simulink subsystem "Encoder_balrob"  (R2024b)
settings: Solver=VariableStepAuto  StartTime=0.0  StopTime=10.0  RelTol=1e-3
values from neighbouring files (symbols this model uses):
  Ts = 1e-2    (= 0.01)    [Plant_balrob_params.m]
undefined symbols (not defined in the file or in its folder): gbox, sens
settings Model: Creator=federico  LastModifiedBy=Riccardo Grosso

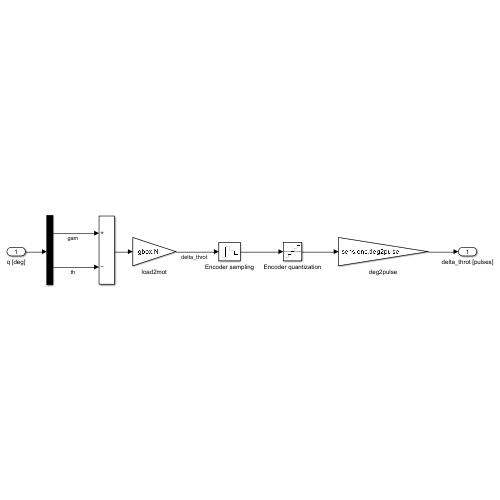
[thumbnail: Simulink's stored preview of the top-level diagram]
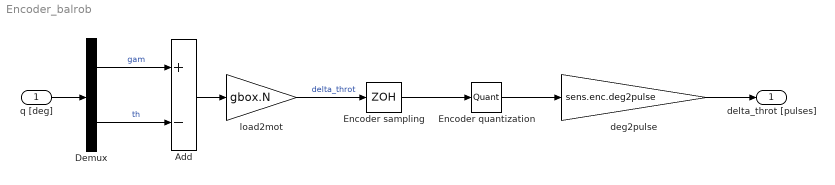
== system Encoder_balrob ==
  q [deg] : Inport
  Add : Sum  Inputs=+-
  Demux : Demux  Outputs=2
  Encoder quantization : Quantizer  QuantizationInterval=sens.enc.pulse2deg
  Encoder sampling : ZeroOrderHold  SampleTime=Ts
  deg2pulse : Gain  Gain=sens.enc.deg2pulse
  load2mot : Gain  Gain=gbox.N
  delta_throt [pulses] : Outport
  wires:
  q [deg]/1 -> Demux/1
  Demux/1 -> Add/1  "gam"
  Demux/2 -> Add/2  "th"
  Add/1 -> load2mot/1
  load2mot/1 -> Encoder sampling/1  "delta_throt"
  Encoder sampling/1 -> Encoder quantization/1
  Encoder quantization/1 -> deg2pulse/1
  deg2pulse/1 -> delta_throt [pulses]/1
